simulink model "trim_model"  (R2025a)
settings: Solver=VariableStepAuto  StartTime=0.0  StopTime=10.0  RelTol=1e-3
values from neighbouring files (symbols this model uses):
  alt = -1000    [Trim_Lin_Lqr.m]
undefined symbols (not defined in the file or in its folder): AngVel, AngVeltr, Coeffs, Lfin, MTOW, R, Rtr, V_i
libraries: aerolibatmos2 x2, matrix_library x2, aerolibobsolete x1, aerolibconvert2 x1
settings Model: Creator=stand-alone1  LastModifiedBy=celal
settings DataIOCC: ExternalInput=getinputstruct(op3)  InitialState=getstatestruct(op3)

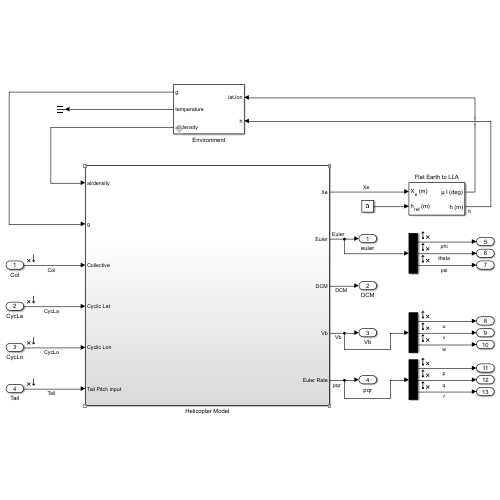
[thumbnail: Simulink's stored preview of the top-level diagram]
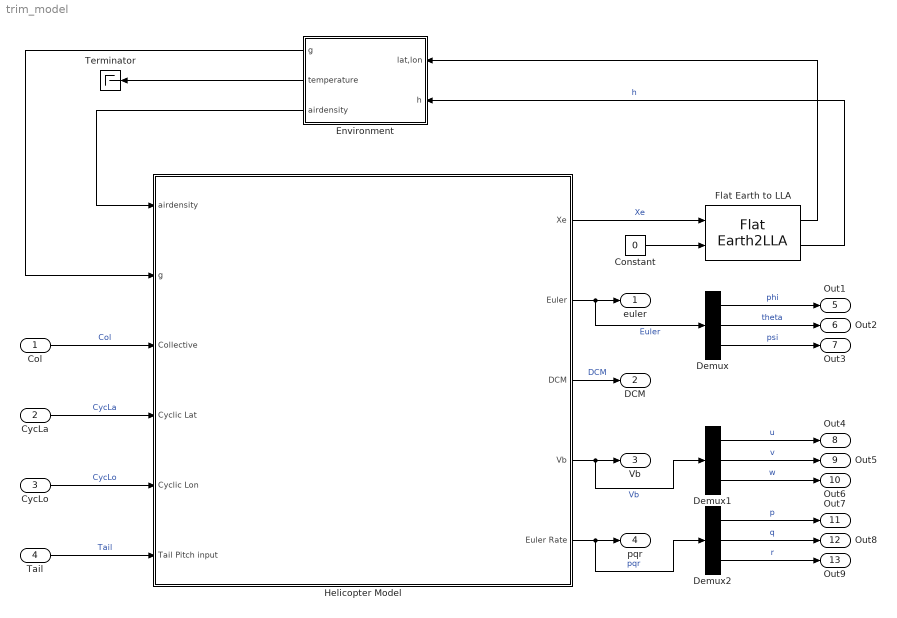
== system trim_model ==
  Col : Inport
  CycLa : Inport  Port=2
  CycLo : Inport  Port=3
  Tail : Inport  Port=4
  Constant : Constant  Value=0
  Demux : Demux  Outputs=3
  Demux1 : Demux  Outputs=3
  Demux2 : Demux  Outputs=3
  Environment : Subsystem  mask{atmomodel=ISA, consg=on}
      mask prompts: atmomodel "Atmosphere Model"; consg "Constant g (Gravitational Acceleration)"
      mask DialogControl a Prompt: Environment
      mask DialogControl b Prompt: Wind simulation, atmosphere properties and gravity model
      mask DialogControl Container4 Prompt: Environment
  Flat Earth to LLA : FlatEarth2LLA  R=6378137
  Helicopter Model : Subsystem
  Terminator : Terminator
  euler : Outport
  DCM : Outport  Port=2
  Vb : Outport  Port=3
  pqr : Outport  Port=4
  Out1 : Outport  Port=5
  Out2 : Outport  Port=6
  Out3 : Outport  Port=7
  Out4 : Outport  Port=8
  Out5 : Outport  Port=9
  Out6 : Outport  Port=10
  Out7 : Outport  Port=11
  Out8 : Outport  Port=12
  Out9 : Outport  Port=13
  wires:
  Flat Earth to LLA/2 -> Environment/2(h)  "h"
  Helicopter Model/1(Xe) -> Flat Earth to LLA/1  "Xe"
  Environment/1(g) -> Helicopter Model/2(g)
  Tail/1 -> Helicopter Model/6(Tail Pitch input)  "Tail"
  Environment/3(airdensity) -> Helicopter Model/1(airdensity)
  Col/1 -> Helicopter Model/3(Collective)  "Col"
  CycLo/1 -> Helicopter Model/5(Cyclic Lon)  "CycLo"
  Flat Earth to LLA/1 -> Environment/1(lat,lon)
  Constant/1 -> Flat Earth to LLA/2
  CycLa/1 -> Helicopter Model/4(Cyclic Lat)  "CycLa"
  Helicopter Model/2(Euler) -> Demux/1, euler/1  "Euler"
  Helicopter Model/3(DCM) -> DCM/1  "DCM"
  Helicopter Model/4(Vb) -> Demux1/1, Vb/1  "Vb"
  Helicopter Model/5(Euler Rate) -> Demux2/1, pqr/1  "pqr"
  Demux2/1 -> Out7/1  "p"
  Demux/2 -> Out2/1  "theta"
  Demux2/2 -> Out8/1  "q"
  Demux2/3 -> Out9/1  "r"
  Demux1/3 -> Out6/1  "w"
  Demux1/2 -> Out5/1  "v"
  Demux1/1 -> Out4/1  "u"
  Demux/1 -> Out1/1  "phi"
  Demux/3 -> Out3/1  "psi"
  Environment/2(temperature) -> Terminator/1

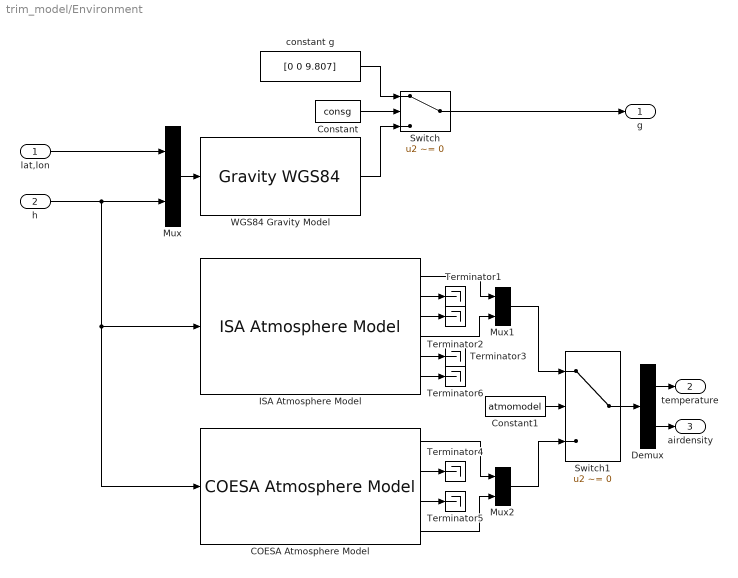
== system trim_model/Environment ==
  lat,lon : Inport
  h : Inport  Port=2
  COESA Atmosphere Model : aerolibatmos2/COESA Atmosphere Model  units=Metric (MKS)  spec=1976 COESA-extended U.S. Standard Atmosphere  model=Profile  profile_var=High temperature  profile_percent=1%  profile_alt=5 km (16404 ft)  envelope_var=High temperature  envelope_percent=1%  action=Warning
  Constant : Constant  Value=consg
  Constant1 : Constant  Value=atmomodel
  Demux : Demux  Outputs=2
  ISA Atmosphere Model : aerolibatmos2/ISA Atmosphere Model  useExtended=off  action=Warning  custom=off  viscosityOut=on  g=9.80665  gamma=1.4  R=287.0531  L=0.0065  h_trop=11000  h_strat=20000  rho0=1.225  P0=101325  T0=288.15  h0=0  S=110.4  Tref=273.15  muref=1.716e-5
  Mux : Mux  Inputs=2
  Mux1 : Mux  Inputs=2
  Mux2 : Mux  Inputs=2
  Switch : Switch  Criteria=u2 ~= 0  SaturateOnIntegerOverflow=off  InputSameDT=off
  Switch1 : Switch  Criteria=u2 ~= 0  SaturateOnIntegerOverflow=off  InputSameDT=off
  Terminator{1..6} (6 alike) : Terminator
  "WGS84 Gravity Model  " : GravityWGS84
  constant g : Constant  Value=[0 0 9.807]
  g : Outport
  temperature : Outport  Port=2
  airdensity : Outport  Port=3
  wires:
  lat,lon/1 -> Mux/1
  Constant/1 -> Switch/2
  constant g/1 -> Switch/1
  "WGS84 Gravity Model  "/1 -> Switch/3
  Switch/1 -> g/1
  Mux/1 -> "WGS84 Gravity Model  "/1
  h/1 -> COESA Atmosphere Model/1, ISA Atmosphere Model/1, Mux/2
  Switch1/1 -> Demux/1
  ISA Atmosphere Model/1 -> Mux1/1
  ISA Atmosphere Model/2 -> Terminator1/1
  ISA Atmosphere Model/3 -> Terminator2/1
  COESA Atmosphere Model/2 -> Terminator4/1
  COESA Atmosphere Model/1 -> Mux2/1
  COESA Atmosphere Model/3 -> Terminator5/1
  ISA Atmosphere Model/4 -> Mux1/2
  COESA Atmosphere Model/4 -> Mux2/2
  Constant1/1 -> Switch1/2
  Mux1/1 -> Switch1/1
  Mux2/1 -> Switch1/3
  Demux/2 -> airdensity/1
  Demux/1 -> temperature/1
  ISA Atmosphere Model/5 -> Terminator3/1
  ISA Atmosphere Model/6 -> Terminator6/1

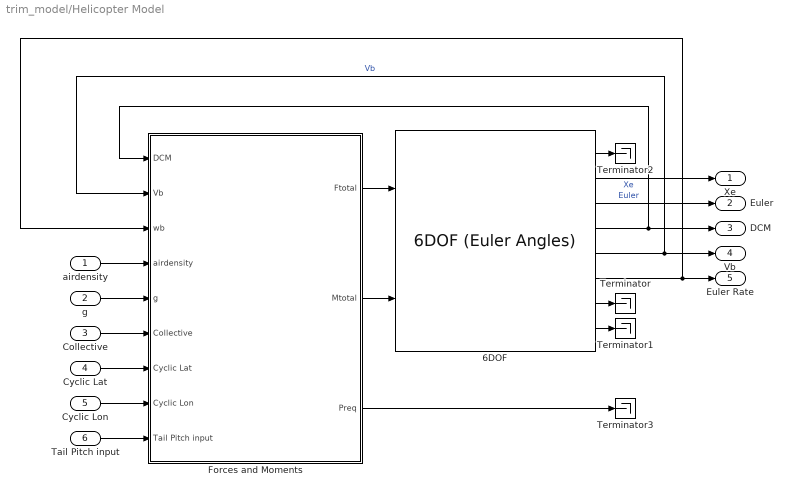
== system trim_model/Helicopter Model ==
  airdensity : Inport
  g : Inport  Port=2
  Collective : Inport  Port=3
  Cyclic Lat : Inport  Port=4
  Cyclic Lon : Inport  Port=5
  Tail Pitch input : Inport  Port=6
  6DOF : aerolibobsolete/6DOF (Euler Angles)  units=Metric (MKS)  mtype=Fixed  rep=Euler Angles  xme_0=[0;0;alt];  Vm_0=[V_i;0;0]  eul_0=[0 0 0]  pm_0=[0 0 0]  mass_0=MTOW  mass_e=0.5  mass_f=2.0  inertia=|  inertia_e=eye(3)  inertia_f=2*eye(3)  k_quat=1.0  vre_flag=off  abi_flag=off  aMode=0  xme_statename=''  Vm_statename=''  eul_statename=''  quat_statename=''  pm_statename=''  mass_statename=''
      | [Inertias(1) 0 0; 0 Inertias(2) 0;
      | 0 0 Inertias(3)];
  Forces and Moments : Subsystem
  Terminator{,1..3} (4 alike) : Terminator
  Xe : Outport
  Euler : Outport  Port=2
  DCM : Outport  Port=3
  Vb : Outport  Port=4
  Euler Rate : Outport  Port=5
  wires:
  6DOF/1 -> Terminator2/1
  6DOF/8 -> Terminator1/1
  Forces and Moments/1(Ftotal) -> 6DOF/1
  Forces and Moments/2(Mtotal) -> 6DOF/2
  6DOF/6 -> Forces and Moments/3(wb), Euler Rate/1
  6DOF/4 -> Forces and Moments/1(DCM), DCM/1
  6DOF/7 -> Terminator/1
  6DOF/5 -> Forces and Moments/2(Vb), Vb/1  "Vb"
  Cyclic Lat/1 -> Forces and Moments/7(Cyclic Lat)
  Collective/1 -> Forces and Moments/6(Collective)
  6DOF/3 -> Euler/1  "Euler"
  Tail Pitch input/1 -> Forces and Moments/9(Tail Pitch input)
  Cyclic Lon/1 -> Forces and Moments/8(Cyclic Lon)
  airdensity/1 -> Forces and Moments/4(airdensity)
  g/1 -> Forces and Moments/5(g)
  6DOF/2 -> Xe/1  "Xe"
  Forces and Moments/3(Preq) -> Terminator3/1

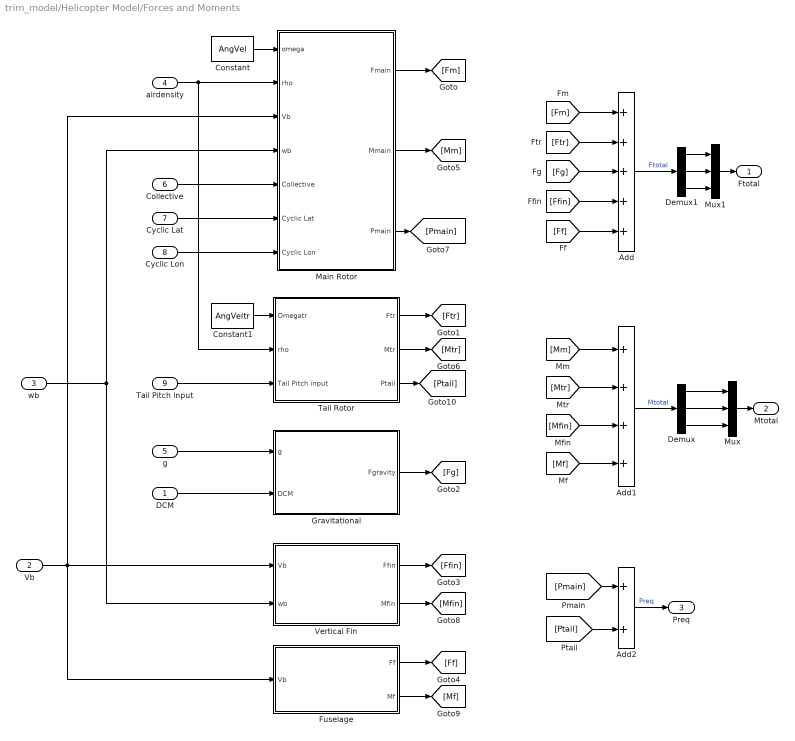
== system trim_model/Helicopter Model/Forces and Moments ==
  DCM : Inport
  Vb : Inport  Port=2
  wb : Inport  Port=3
  airdensity : Inport  Port=4
  g : Inport  Port=5
  Collective : Inport  Port=6
  Cyclic Lat : Inport  Port=7
  Cyclic Lon : Inport  Port=8
  Tail Pitch input : Inport  Port=9
  Add : Sum  Inputs=+++++
  Add1 : Sum  Inputs=++++
  Add2 : Sum
  Constant : Constant  Value=AngVel
  Constant1 : Constant  Value=AngVeltr
  Demux : Demux  Outputs=3
  Demux1 : Demux  Outputs=3
  Fuselage : Subsystem
  Gravitational : Subsystem
  Main Rotor : Subsystem
  Mux : Mux  Inputs=3
  Mux1 : Mux  Inputs=3
  Tail Rotor : Subsystem
  Vertical Fin : Subsystem
  Ftotal : Outport
  Mtotal : Outport  Port=2
  Preq : Outport  Port=3
  wires:
  Add/1 -> Demux1/1  "Ftotal"
  Add1/1 -> Demux/1  "Mtotal"
  Main Rotor/1(Fmain) -> [Fm]
  Tail Rotor/1(Ftr) -> [Ftr]
  Gravitational/1(Fgravity) -> [Fg]
  Vertical Fin/1(Ffin) -> [Ffin]
  [Fm] -> Add/1
  [Ftr] -> Add/2
  [Fg] -> Add/3
  [Ffin] -> Add/4
  [Ff] -> Add/5
  Main Rotor/2(Mmain) -> [Mm]
  Tail Rotor/2(Mtr) -> [Mtr]
  Vertical Fin/2(Mfin) -> [Mfin]
  [Mm] -> Add1/1
  [Mtr] -> Add1/2
  [Mf] -> Add1/4
  [Mfin] -> Add1/3
  Constant/1 -> Main Rotor/1(omega)
  Constant1/1 -> Tail Rotor/1(Omegatr)
  airdensity/1 -> Tail Rotor/2(rho), Main Rotor/2(rho)
  g/1 -> Gravitational/1(g)
  DCM/1 -> Gravitational/2(DCM)
  Collective/1 -> Main Rotor/5(Collective)
  Tail Pitch input/1 -> Tail Rotor/3(Tail Pitch input)
  Cyclic Lat/1 -> Main Rotor/6(Cyclic Lat)
  Cyclic Lon/1 -> Main Rotor/7(Cyclic Lon)
  wb/1 -> Main Rotor/4(wb), Vertical Fin/2(wb)
  Vb/1 -> Fuselage/1(Vb), Main Rotor/3(Vb), Vertical Fin/1(Vb)
  Add2/1 -> Preq/1  "Preq"
  Main Rotor/3(Pmain) -> [Pmain]
  Tail Rotor/3(Ptail) -> [Ptail]
  [Pmain] -> Add2/1
  [Ptail] -> Add2/2
  Fuselage/1(Ff) -> [Ff]
  Fuselage/2(Mf) -> [Mf]
  Mux/1 -> Mtotal/1
  Mux1/1 -> Ftotal/1
  Demux/3 -> Mux/3
  Demux/2 -> Mux/2
  Demux1/1 -> Mux1/1
  Demux1/2 -> Mux1/2
  Demux1/3 -> Mux1/3
  Demux/1 -> Mux/1

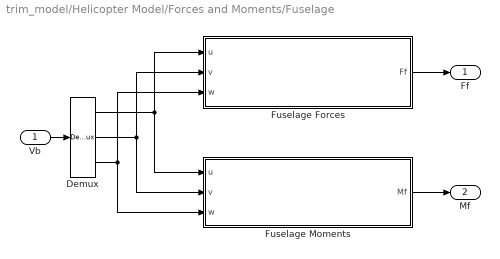
== system trim_model/Helicopter Model/Forces and Moments/Fuselage ==
  Vb : Inport
  Demux : Demux  Outputs=3
  Fuselage Forces : Subsystem
  Fuselage Moments : Subsystem
  Ff : Outport
  Mf : Outport  Port=2
  wires:
  Demux/1 -> Fuselage Forces/1(u), Fuselage Moments/1(u)
  Demux/2 -> Fuselage Moments/2(v), Fuselage Forces/2(v)
  Demux/3 -> Fuselage Moments/3(w), Fuselage Forces/3(w)
  Vb/1 -> Demux/1
  Fuselage Moments/1(Mf) -> Mf/1
  Fuselage Forces/1(Ff) -> Ff/1

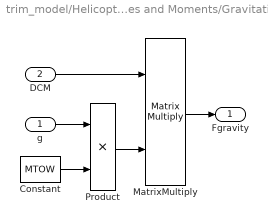
== system trim_model/Helicopter Model/Forces and Moments/Gravitational ==
  g : Inport
  DCM : Inport  Port=2
  Constant : Constant  Value=MTOW
  MatrixMultiply : Product  Multiplication=Matrix(*)
  Product : Product
  Fgravity : Outport
  wires:
  DCM/1 -> MatrixMultiply/1
  MatrixMultiply/1 -> Fgravity/1
  Product/1 -> MatrixMultiply/2
  Constant/1 -> Product/2
  g/1 -> Product/1

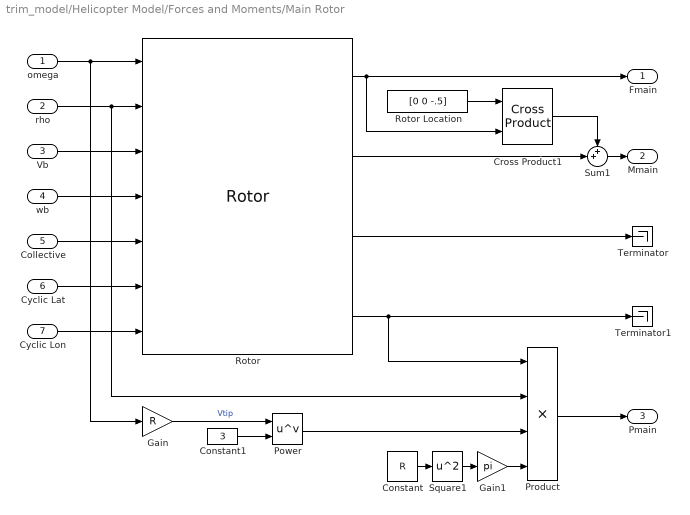
== system trim_model/Helicopter Model/Forces and Moments/Main Rotor ==
  omega : Inport
  rho : Inport  Port=2
  Vb : Inport  Port=3
  wb : Inport  Port=4
  Collective : Inport  Port=5
  Cyclic Lat : Inport  Port=6
  Cyclic Lon : Inport  Port=7
  Constant : Constant  Value=R
  Constant1 : Constant  Value=3
  Cross Product1 : matrix_library/Cross Product
  Gain : Gain  Gain=R
  Gain1 : Gain  Gain=pi
  Power : Math  Operator=pow
  Product : Product  Inputs=4
  Rotor : Rotor  modelMode=With flap effects  controlInput=on  CTCQMode=Compute using BEMT  Nb=Nb  CTout=on  radius=R  chord=c  clalpha=CL_a  cd0=0.009  gamma=lockNum  thetaRoot=rootang  thetaTwist=twistang
  Rotor Location : Constant  Value=[0 0 -.5]  VectorParams1D=off
  Square1 : Math  Operator=square
  Sum1 : Sum  Inputs=++|
  Terminator : Terminator
  Terminator1 : Terminator
  Fmain : Outport
  Mmain : Outport  Port=2
  Pmain : Outport  Port=3
  wires:
  omega/1 -> Gain/1, Rotor/1
  rho/1 -> Rotor/2, Product/2
  Rotor/3 -> Terminator/1
  Rotor/4 -> Terminator1/1, Product/1
  Cyclic Lon/1 -> Rotor/7
  Cyclic Lat/1 -> Rotor/6
  Vb/1 -> Rotor/3
  wb/1 -> Rotor/4
  Power/1 -> Product/3
  Gain/1 -> Power/1  "Vtip"
  Constant/1 -> Square1/1
  Square1/1 -> Gain1/1
  Gain1/1 -> Product/4
  Constant1/1 -> Power/2
  Product/1 -> Pmain/1
  Sum1/1 -> Mmain/1
  Rotor/1 -> Cross Product1/2, Fmain/1
  Rotor/2 -> Sum1/2
  Collective/1 -> Rotor/5
  Cross Product1/1 -> Sum1/1
  Rotor Location/1 -> Cross Product1/1

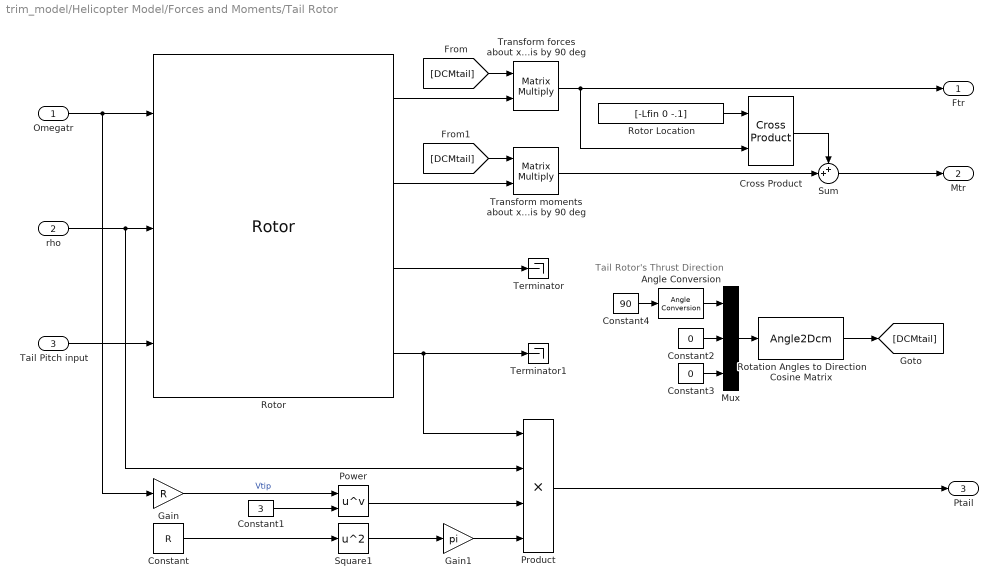
== system trim_model/Helicopter Model/Forces and Moments/Tail Rotor ==
  note: Tail Rotor's Thrust Direction
  Omegatr : Inport
  rho : Inport  Port=2
  Tail Pitch input : Inport  Port=3
  Angle Conversion : aerolibconvert2/Angle Conversion  IU=deg  OU=rad
  Constant : Constant  Value=R
  Constant1 : Constant  Value=3
  Constant2 : Constant  Value=0
  Constant3 : Constant  Value=0
  Constant4 : Constant  Value=90
  Cross Product : matrix_library/Cross Product
  Gain : Gain  Gain=R
  Gain1 : Gain  Gain=pi
  Mux : Mux  Inputs=3
  Power : Math  Operator=pow
  Product : Product  Inputs=4
  Rotation Angles to Direction Cosine Matrix : Angle2Dcm  rotationOrder=XYZ
      settings: AttributesFormatString=Rotation Order: %<rotationOrder>
  Rotor : Rotor  controlInput=on  CTCQMode=Compute using BEMT  Nb=Nbtr  CTout=on  radius=Rtr+.1  chord=0.12  cd0=0.009  thetaRoot=0.0001  thetaTwist=0.0001
  Rotor Location : Constant  Value=[-Lfin 0 -.1]  VectorParams1D=off
  Square1 : Math  Operator=square
  Sum : Sum  Inputs=++|
  Terminator : Terminator
  Terminator1 : Terminator
  "Transform forces about x-axis by 90 deg " : Product  Multiplication=Matrix(*)
  Transform moments about x-axis by 90 deg : Product  Multiplication=Matrix(*)
  Ftr : Outport
  Mtr : Outport  Port=2
  Ptail : Outport  Port=3
  wires:
  Rotor/3 -> Terminator/1
  Tail Pitch input/1 -> Rotor/3
  Power/1 -> Product/3
  Constant1/1 -> Power/2
  Gain/1 -> Power/1  "Vtip"
  rho/1 -> Product/2, Rotor/2
  Rotor/4 -> Product/1, Terminator1/1
  Gain1/1 -> Product/4
  Omegatr/1 -> Gain/1, Rotor/1
  Square1/1 -> Gain1/1
  Constant/1 -> Square1/1
  Product/1 -> Ptail/1
  Rotor/2 -> Transform moments about x-axis by 90 deg/2
  Sum/1 -> Mtr/1
  Rotor Location/1 -> Cross Product/1
  Constant4/1 -> Angle Conversion/1
  Transform moments about x-axis by 90 deg/1 -> Sum/2
  Mux/1 -> Rotation Angles to Direction Cosine Matrix/1
  Angle Conversion/1 -> Mux/1
  Constant2/1 -> Mux/2
  Rotor/1 -> "Transform forces about x-axis by 90 deg "/2
  "Transform forces about x-axis by 90 deg "/1 -> Cross Product/2, Ftr/1
  Cross Product/1 -> Sum/1
  Constant3/1 -> Mux/3
  Rotation Angles to Direction Cosine Matrix/1 -> [DCMtail]
  [DCMtail] -> "Transform forces about x-axis by 90 deg "/1
  [DCMtail] -> Transform moments about x-axis by 90 deg/1

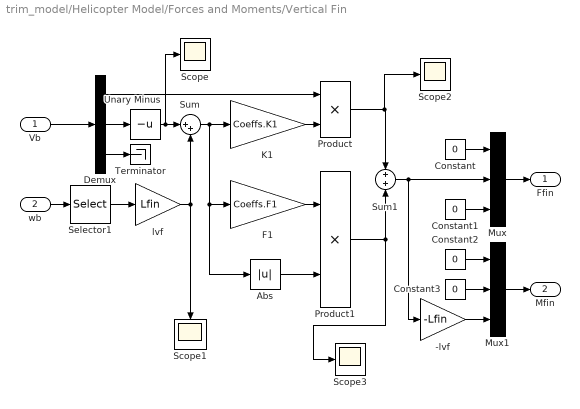
== system trim_model/Helicopter Model/Forces and Moments/Vertical Fin ==
  Vb : Inport
  wb : Inport  Port=2
  -lvf : Gain  Gain=-Lfin
  Abs : Abs  SaturateOnIntegerOverflow=off
  Constant{,1..3} (4 alike) : Constant  Value=0
  Demux : Demux  Outputs=3
  F1 : Gain  Gain=Coeffs.F1
  K1 : Gain  Gain=Coeffs.K1
  Mux : Mux  Inputs=3
  Mux1 : Mux  Inputs=3
  Product : Product
  Product1 : Product
  Scope{,1..3} (4 alike) : Scope
      Scope settings: ActiveDisplayYMinimum=-0.16634  ActiveDisplayYMaximum=1.49709
      Scope1 settings: ActiveDisplayYMinimum=-1.37396  ActiveDisplayYMaximum=0.15266  DataLoggingVariableName=ScopeData2
      Scope2 settings: ActiveDisplayYMinimum=-4.1E-7  ActiveDisplayYMaximum=8E-8  DataLoggingVariableName=ScopeData3
      Scope3 settings: ActiveDisplayYMinimum=-7.6E-9  ActiveDisplayYMaximum=8E-10  DataLoggingVariableName=ScopeData4
  Selector1 : Selector  InputPortWidth=3  IndexOptions=Index vector (dialog)  Indices=[3]  OutputSizes=1
  Sum : Sum  Inputs=|++
  Sum1 : Sum  Inputs=+|+
  Terminator : Terminator
  Unary Minus : UnaryMinus
  lvf : Gain  Gain=Lfin
  Ffin : Outport
  Mfin : Outport  Port=2
  wires:
  Vb/1 -> Demux/1
  Unary Minus/1 -> Scope/1, Sum/1
  wb/1 -> Selector1/1
  Selector1/1 -> lvf/1
  lvf/1 -> Scope1/1, Sum/2
  Demux/2 -> Unary Minus/1
  Demux/1 -> Product/1
  K1/1 -> Product/2
  F1/1 -> Product1/1
  Sum/1 -> F1/1, Abs/1, K1/1
  Abs/1 -> Product1/2
  Demux/3 -> Terminator/1
  Mux/1 -> Ffin/1
  Mux1/1 -> Mfin/1
  Constant/1 -> Mux/1
  Constant1/1 -> Mux/3
  Constant3/1 -> Mux1/2
  Constant2/1 -> Mux1/1
  Product/1 -> Scope2/1, Sum1/1
  Product1/1 -> Scope3/1, Sum1/2
  Sum1/1 -> -lvf/1, Mux/2
  -lvf/1 -> Mux1/3

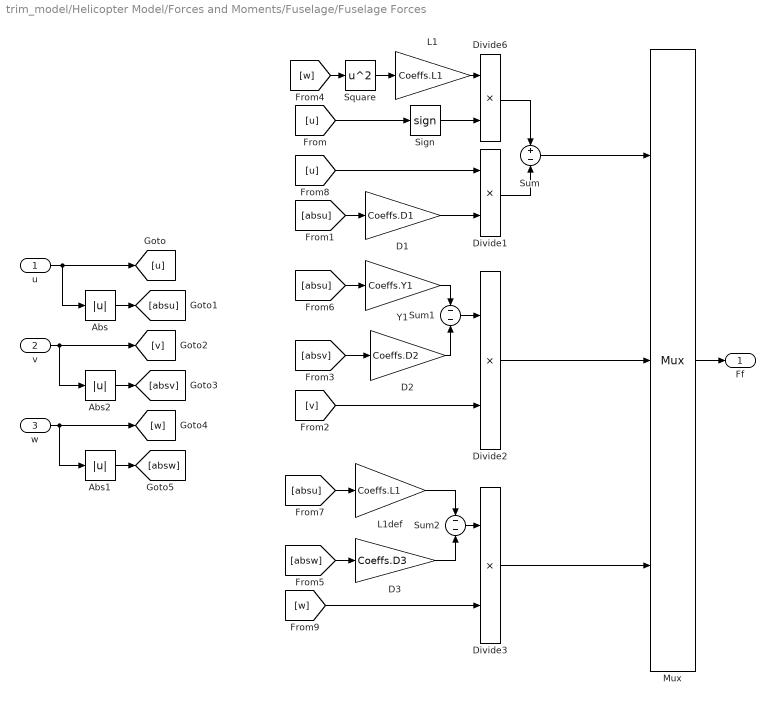
== system trim_model/Helicopter Model/Forces and Moments/Fuselage/Fuselage Forces ==
  u : Inport
  v : Inport  Port=2
  w : Inport  Port=3
  Abs : Abs  SaturateOnIntegerOverflow=off
  Abs1 : Abs  SaturateOnIntegerOverflow=off
  Abs2 : Abs  SaturateOnIntegerOverflow=off
  D1 : Gain  Gain=Coeffs.D1
  D2 : Gain  Gain=Coeffs.D2
  D3 : Gain  Gain=Coeffs.D3
  Divide{1..3,6} (4 alike) : Product  Inputs=**
  L1 : Gain  Gain=Coeffs.L1
  L1def : Gain  Gain=Coeffs.L1
  Mux : Mux  Inputs=3
  Sign : Signum
  Square : Math  Operator=square
  Sum : Sum  Inputs=+|-
  Sum1 : Sum  Inputs=-|-
  Sum2 : Sum  Inputs=-|-
  Y1 : Gain  Gain=Coeffs.Y1
  Ff : Outport
  wires:
  Sign/1 -> Divide6/2
  D2/1 -> Sum1/2
  Sum1/1 -> Divide2/1
  Divide6/1 -> Sum/1
  Divide2/1 -> Mux/2
  D3/1 -> Sum2/2
  L1def/1 -> Sum2/1
  Divide1/1 -> Sum/2
  Y1/1 -> Sum1/1
  Square/1 -> L1/1
  L1/1 -> Divide6/1
  Sum/1 -> Mux/1
  Divide3/1 -> Mux/3
  Sum2/1 -> Divide3/1
  Mux/1 -> Ff/1
  D1/1 -> Divide1/2
  [absu] -> D1/1
  [absu] -> Y1/1
  [absu] -> L1def/1
  [u] -> Sign/1
  [u] -> Divide1/1
  u/1 -> [u], Abs/1
  Abs/1 -> [absu]
  [w] -> Square/1
  [w] -> Divide3/2
  [absw] -> D3/1
  w/1 -> [w], Abs1/1
  Abs1/1 -> [absw]
  [v] -> Divide2/2
  [absv] -> D2/1
  v/1 -> [v], Abs2/1
  Abs2/1 -> [absv]

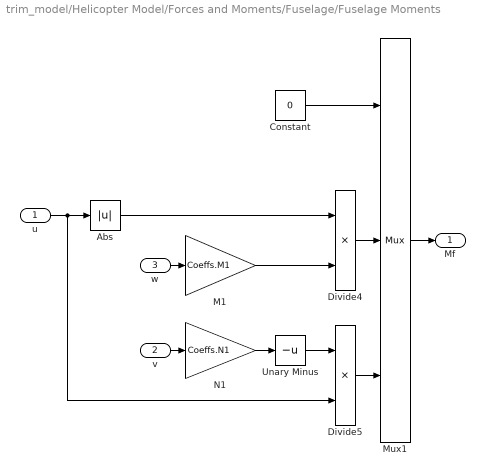
== system trim_model/Helicopter Model/Forces and Moments/Fuselage/Fuselage Moments ==
  u : Inport
  v : Inport  Port=2
  w : Inport  Port=3
  Abs : Abs  SaturateOnIntegerOverflow=off
  Constant : Constant  Value=0
  Divide4 : Product  Inputs=**
  Divide5 : Product  Inputs=**
  M1 : Gain  Gain=Coeffs.M1
  Mux1 : Mux  Inputs=3
  N1 : Gain  Gain=Coeffs.N1
  Unary Minus : UnaryMinus
  Mf : Outport
  wires:
  u/1 -> Divide5/2, Abs/1
  M1/1 -> Divide4/2
  N1/1 -> Unary Minus/1
  Mux1/1 -> Mf/1
  Divide5/1 -> Mux1/3
  Constant/1 -> Mux1/1
  v/1 -> N1/1
  Unary Minus/1 -> Divide5/1
  Divide4/1 -> Mux1/2
  w/1 -> M1/1
  Abs/1 -> Divide4/1
